simulink model "Model_leis_de_Newton"  (R2018a)
settings: Solver=FixedStepAuto  StartTime=0.0  StopTime=130  FixedStep=0.001  RelTol=1e-3
values from neighbouring files (symbols this model uses):
  C = [1 0 0 0 ... (first row only)    [Dados.m]    (also in Dados_correct.m; Function_ARE.m = D; teste.m = D)
  c = 0.0076    [Dados.m]    (also in Dados_correct.m; Function_ARE.m; areklmn_reactor.m; fd0.m)
  g = 9.81    [Dados.m]    (also in Dados_correct.m; Function_ARE.m; areklmn_reactor.m; fd0.m)
  Jphi = 0.00201    [Dados.m]    (also in Dados_correct.m; Function_ARE.m; areklmn_reactor.m; fd0.m)
  Jteta = 0.005425    [Dados.m]    (also in Dados_correct.m; Function_ARE.m; areklmn_reactor.m; fd0.m)
  K1 = Kpi(:,1:4)    [Dados.m]    (also in Dados_correct.m = Kpi90(:,1:4); Function_ARE.m = K(:,1:4); teste.m = K(:,1:4))
  K1_30 = Kpi30(:,1:4)    [Dados_correct.m]
  K2 = Kpi(:,5:6)    [Dados.m]    (also in Dados_correct.m = Kpi90(:,5:6); Function_ARE.m = K(:,5:6); teste.m = K(:,5:6))
  K2_30 = Kpi30(:,5:6)    [Dados_correct.m]
  Kf = 0.0275    [Dados.m]    (also in Dados_correct.m = 0.06; Function_ARE.m = 0.056; areklmn_reactor.m = 0.056; fd0.m = 0.056)
  L1 = 0.3    [Dados.m]    (also in Dados_correct.m = 0.227; Function_ARE.m = 0.227; areklmn_reactor.m = 0.227; fd0.m = 0.227)
  L2 = 0.1    [Dados.m]    (also in Dados_correct.m = 0.08; Function_ARE.m = 0.08; areklmn_reactor.m = 0.08; fd0.m = 0.08)
  Lw = 0.13    [Dados_correct.m]    (also in Function_ARE.m = 0.15; areklmn_reactor.m = 0.15; fd0.m = 0.15; teste.m = 0.15)
  Mh = 0.08    [Dados.m]    (also in Dados_correct.m; Function_ARE.m; areklmn_reactor.m; fd0.m)
  Mw = 0.08    [Dados_correct.m]    (also in Function_ARE.m = 0.039; areklmn_reactor.m = 0.039; fd0.m = 0.039; teste.m = 0.039)
undefined symbols (not defined in the file or in its folder): DiscIntNeverNeededParam, K1_130, K1_150, K1_90, K2_130, K2_150, K2_90, sigbuilder_block
settings Model: Creator=stayn  LastModifiedBy=stayn

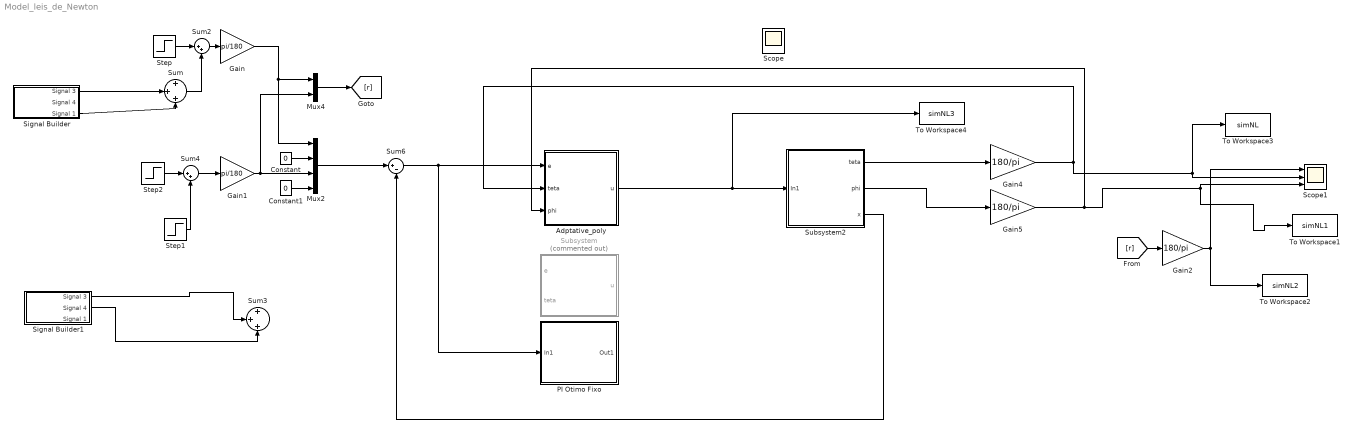
== system Model_leis_de_Newton ==
  Adptative_poly : Subsystem
  Constant : Constant  Value=0
  Constant1 : Constant  Value=0
  Gain : Gain  Gain=pi/180
  Gain1 : Gain  Gain=pi/180
  Gain2 : Gain  Gain=180/pi
  Gain4 : Gain  Gain=180/pi
  Gain5 : Gain  Gain=180/pi
  Mux2 : Mux
  Mux4 : Mux  Inputs=2
  PI Otimo Fixo : Subsystem
  Scope : Scope  NumInputPorts=2
  Scope1 : Scope  NumInputPorts=3
  Signal Builder : Subsystem  Tag=STV Subsys  LoadFcn=sigbuilder_block('load');  StartFcn=sigbuilder_block('start');  StopFcn=sigbuilder_block('stop');  ClipboardFcn=sigbuilder_block('clipboard');  mask(Sigbuilder block){tuvar=[0:10]}
      mask help: Simulink:masks:SigbuilderBlock_MD
      mask init:
      | if ~strcmp(get_param(bdroot(gcbh),'SimulationStatus'),'stopped') tuvar = sigbuilder_block('maskInit'); end
      settings: CopyFcn=sigbuilder_block('copy');  DeleteFcn=sigbuilder_block('delete');  ModelCloseFcn=sigbuilder_block('modelClose');  PreSaveFcn=sigbuilder_block('preSave');  PauseFcn=sigbuilder_block('pause');  ContinueFcn=sigbuilder_block('continue');  NameChangeFcn=sigbuilder_block('namechange');  OpenFcn=sigbuilder_block('open',[6 30 1012.5 447.75 ]);  CloseFcn=sigbuilder_block('close');
      mask Display: plot(0, 0, 100, 100,[2, 2, 32, 32, 2], [68, 8, 8, 68, 68],[32, 2], [38, 38], [32, 19, 2],[53, 60, 44], [32, 17, 17, 2],[16, 16, 31, 31]);txt = getActiveGroup(gcbh);text(2, 100, txt,'verticalAlignment', 'top');
  Signal Builder1 : Subsystem  Tag=STV Subsys  LoadFcn=sigbuilder_block('load');  StartFcn=sigbuilder_block('start');  StopFcn=sigbuilder_block('stop');  ClipboardFcn=sigbuilder_block('clipboard');  mask(Sigbuilder block){tuvar=[0:10]}
      mask help: Simulink:masks:SigbuilderBlock_MD
      mask init:
      | if ~strcmp(get_param(bdroot(gcbh),'SimulationStatus'),'stopped') tuvar = sigbuilder_block('maskInit'); end
      settings: CopyFcn=sigbuilder_block('copy');  DeleteFcn=sigbuilder_block('delete');  ModelCloseFcn=sigbuilder_block('modelClose');  PreSaveFcn=sigbuilder_block('preSave');  PauseFcn=sigbuilder_block('pause');  ContinueFcn=sigbuilder_block('continue');  NameChangeFcn=sigbuilder_block('namechange');  OpenFcn=sigbuilder_block('open',[6 30 1006.5 447.75 ]);  CloseFcn=sigbuilder_block('close');
      mask Display: plot(0, 0, 100, 100,[2, 2, 32, 32, 2], [68, 8, 8, 68, 68],[32, 2], [38, 38], [32, 19, 2],[53, 60, 44], [32, 17, 17, 2],[16, 16, 31, 31]);txt = getActiveGroup(gcbh);text(2, 100, txt,'verticalAlignment', 'top');
  Step : Step  Time=0  After=90  SampleTime=0
  Step1 : Step  Time=120  After=-20  SampleTime=0
  Step2 : Step  Time=100  After=30  SampleTime=0
  Subsystem : Subsystem  Commented=on
  Subsystem2 : Subsystem
  Sum : Sum  Inputs=+|+|+
  Sum2 : Sum  Inputs=|++
  Sum3 : Sum  Inputs=+|+|+
  Sum4 : Sum  Inputs=|++
  Sum6 : Sum  Inputs=|+-
  To Workspace1 : ToWorkspace  VariableName=simNL1  SampleTime=0.001
      settings: Save2DSignal=2-D array (concatenate along first dimension)
  To Workspace2 : ToWorkspace  VariableName=simNL2  SampleTime=0.001
      settings: Save2DSignal=2-D array (concatenate along first dimension)
  To Workspace3 : ToWorkspace  VariableName=simNL  SaveFormat=Structure With Time  SampleTime=0.001
      settings: Save2DSignal=2-D array (concatenate along first dimension)
  To Workspace4 : ToWorkspace  VariableName=simNL3  SampleTime=0.001
      settings: Save2DSignal=2-D array (concatenate along first dimension)
  wires:
  Subsystem2/3("x ") -> Sum6/2
  Sum6/1 -> PI Otimo Fixo/1(In1), Adptative_poly/1(e)
  Subsystem2/1("teta ") -> Gain4/1
  Signal Builder1/2(Signal 4) -> Sum3/3
  Sum4/1 -> Gain1/1
  Step2/1 -> Sum4/1
  Signal Builder1/1(Signal 3) -> Sum3/2
  Signal Builder/1(Signal 3) -> Sum/2
  Step/1 -> Sum2/1
  Mux2/1 -> Sum6/1
  Sum2/1 -> Gain/1
  Mux4/1 -> [r]
  Constant/1 -> Mux2/2
  Gain1/1 -> Mux4/2, Mux2/3
  Gain/1 -> Mux2/1, Mux4/1
  Constant1/1 -> Mux2/4
  [r] -> Gain2/1
  Signal Builder/3(Signal 1) -> Sum/3
  Gain2/1 -> To Workspace2/1, Scope1/1
  Gain5/1 -> Adptative_poly/3("phi "), To Workspace1/1, Scope1/3
  Subsystem2/2(phi) -> Gain5/1
  Gain4/1 -> To Workspace3/1, Scope1/2, Adptative_poly/2(teta)
  Adptative_poly/1(u) -> To Workspace4/1, Subsystem2/1(In1)
  Step1/1 -> Sum4/2
  Sum/1 -> Sum2/2

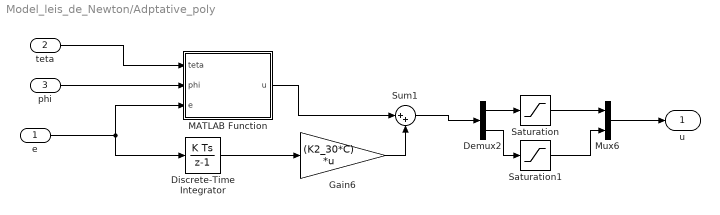
== system Model_leis_de_Newton/Adptative_poly ==
  e : Inport
  teta : Inport  Port=2
  "phi " : Inport  Port=3
  Demux2 : Demux  Outputs=2
  Discrete-Time Integrator : DiscreteIntegrator  SampleTime=0.001  ICPrevOutput=DiscIntNeverNeededParam  ICPrevScaledInput=DiscIntNeverNeededParam
  Gain6 : Gain  Gain=(K2_30*C)  Multiplication=Matrix(K*u) (u vector)
  MATLAB Function : MATLAB Function  TreatAsAtomicUnit=on
  Mux6 : Mux  Inputs=2
  Saturation : Saturate  UpperLimit=10  LowerLimit=0
  Saturation1 : Saturate  UpperLimit=5  LowerLimit=-5
  Sum1 : Sum  Inputs=|++
  u : Outport
  wires:
  MATLAB Function/1(u) -> Sum1/1
  e/1 -> Discrete-Time Integrator/1, MATLAB Function/3(e)
  Demux2/1 -> Saturation/1
  Saturation1/1 -> Mux6/2
  Demux2/2 -> Saturation1/1
  Discrete-Time Integrator/1 -> Gain6/1
  Gain6/1 -> Sum1/2
  teta/1 -> MATLAB Function/1(teta)
  Sum1/1 -> Demux2/1
  Saturation/1 -> Mux6/1
  Mux6/1 -> u/1
  "phi "/1 -> MATLAB Function/2(phi)

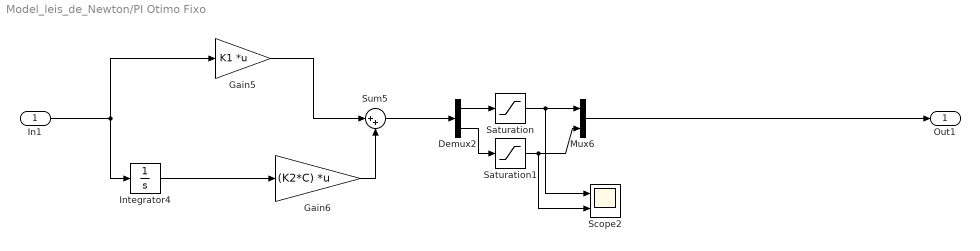
== system Model_leis_de_Newton/PI Otimo Fixo ==
  In1 : Inport
  Demux2 : Demux  Outputs=2
  Gain5 : Gain  Gain=K1  Multiplication=Matrix(K*u) (u vector)
  Gain6 : Gain  Gain=(K2*C)  Multiplication=Matrix(K*u) (u vector)
  Integrator4 : Integrator
  Mux6 : Mux  Inputs=2
  Saturation : Saturate  UpperLimit=10  LowerLimit=0
  Saturation1 : Saturate  UpperLimit=5  LowerLimit=-5
  Scope2 : Scope  NumInputPorts=2
  Sum5 : Sum  Inputs=|++
  Out1 : Outport
  wires:
  Saturation/1 -> Scope2/1, Mux6/1
  Integrator4/1 -> Gain6/1
  Demux2/1 -> Saturation/1
  Gain6/1 -> Sum5/2
  In1/1 -> Gain5/1, Integrator4/1
  Gain5/1 -> Sum5/1
  Saturation1/1 -> Mux6/2, Scope2/2
  Demux2/2 -> Saturation1/1
  Sum5/1 -> Demux2/1
  Mux6/1 -> Out1/1

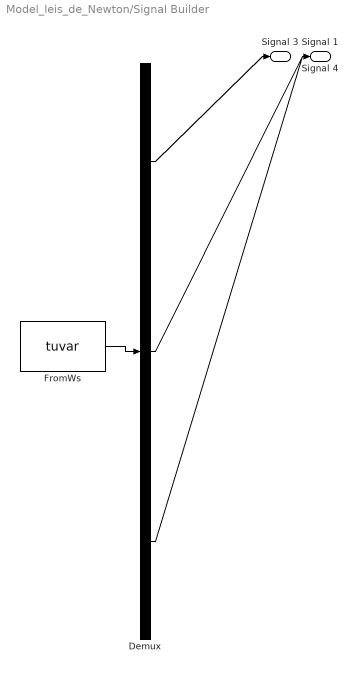
== system Model_leis_de_Newton/Signal Builder ==
  Demux : Demux  Tag=STV Demux  Outputs=3
  FromWs : FromWorkspace  Tag=STV FromWs  VariableName=tuvar  SampleTime=0
      SigBuilderData=|
      | common.afterFinalStr = 'Extrapolate'
      | common.sampleTime = 0
      | dataSet.timeRange = [0 100]
      | dataSet.name = 'Group 1'
      | sbobj.Groups.Name = 'Group 1'
      | sbobj.Groups.Signals(1).Name = 'Signal 3'
      | sbobj.Groups.Signals(1).XData = [0 20 20 45 45 100]
      | sbobj.Groups.Signals(1).YData = [0 0 45 45 0 0]
      | sbobj.Groups.Signals(2).Name = 'Signal 4'
      | sbobj.Groups.Signals(2).XData = [0 65 65 100]
      | sbobj.Groups.Signals(2).YData = [0 0 -35 -35]
      | sbobj.Groups.Signals(3).Name = 'Signal 1'
      | sbobj.Groups.Signals(3).XData = [0 65 65 85 85 100]
      | sbobj.Groups.Signals(3).YData = [0 0 -30 -30 0 0]
      | sbobj.Groups.TimeRange = [0 100]
  Signal 3 : Outport  Tag=STV Outport
  Signal 4 : Outport  Tag=STV Outport  Port=2
  Signal 1 : Outport  Tag=STV Outport  Port=3
  wires:
  FromWs/1 -> Demux/1
  Demux/1 -> Signal 3/1
  Demux/2 -> Signal 4/1
  Demux/3 -> Signal 1/1

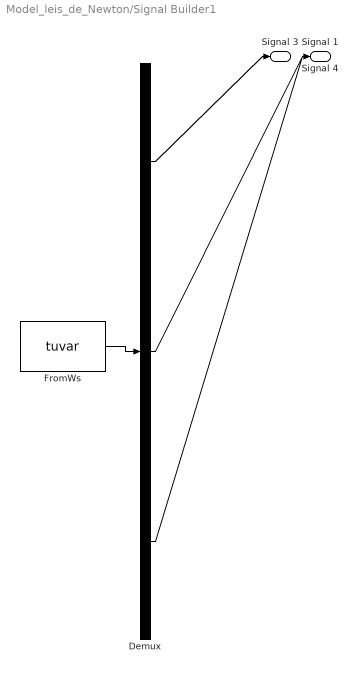
== system Model_leis_de_Newton/Signal Builder1 ==
  Demux : Demux  Tag=STV Demux  Outputs=3
  FromWs : FromWorkspace  Tag=STV FromWs  VariableName=tuvar  SampleTime=0
      SigBuilderData=|
      | common.afterFinalStr = 'Extrapolate'
      | common.sampleTime = 0
      | dataSet.timeRange = [0 100]
      | dataSet.name = 'Group 1'
      | sbobj.Groups.Name = 'Group 1'
      | sbobj.Groups.Signals(1).Name = 'Signal 3'
      | sbobj.Groups.Signals(1).XData = [0 15.1 15.1 30.1 30.1 100]
      | sbobj.Groups.Signals(1).YData = [0 0 -45 -45 0 0]
      | sbobj.Groups.Signals(2).Name = 'Signal 4'
      | sbobj.Groups.Signals(2).XData = [0 45 45 60 60 100]
      | sbobj.Groups.Signals(2).YData = [0 0 40 40 0 0]
      | sbobj.Groups.Signals(3).Name = 'Signal 1'
      | sbobj.Groups.Signals(3).XData = [0 70.1 70.1 85.6 85.6 100]
      | sbobj.Groups.Signals(3).YData = [0 0 50.5 50.5 0 0]
      | sbobj.Groups.TimeRange = [0 100]
  Signal 3 : Outport  Tag=STV Outport
  Signal 4 : Outport  Tag=STV Outport  Port=2
  Signal 1 : Outport  Tag=STV Outport  Port=3
  wires:
  FromWs/1 -> Demux/1
  Demux/1 -> Signal 3/1
  Demux/2 -> Signal 4/1
  Demux/3 -> Signal 1/1

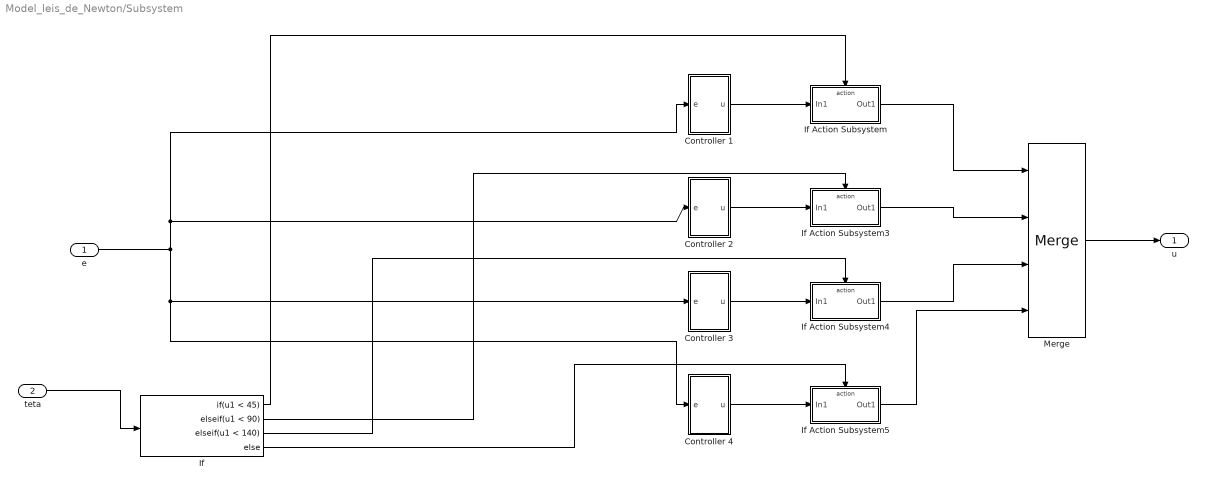
== system Model_leis_de_Newton/Subsystem ==
  e : Inport
  teta : Inport  Port=2
  Controller 1 : Subsystem
  Controller 2 : Subsystem
  Controller 3 : Subsystem
  Controller 4 : Subsystem
  If : If  IfExpression=u1 < 45  ElseIfExpressions=u1 < 90, u1 < 140
  If Action Subsystem : Subsystem  TreatAsAtomicUnit=on
  If Action Subsystem3 : Subsystem  TreatAsAtomicUnit=on
  If Action Subsystem4 : Subsystem  TreatAsAtomicUnit=on
  If Action Subsystem5 : Subsystem  TreatAsAtomicUnit=on
  Merge : Merge  Inputs=4
  u : Outport
  wires:
  Controller 3/1("u ") -> If Action Subsystem4/1(In1)
  Controller 1/1("u ") -> If Action Subsystem/1(In1)
  e/1 -> Controller 1/1("e "), Controller 2/1("e "), Controller 4/1("e "), Controller 3/1("e ")
  If Action Subsystem4/1(Out1) -> Merge/3
  teta/1 -> If/1
  Merge/1 -> u/1
  Controller 4/1("u ") -> If Action Subsystem5/1(In1)
  If Action Subsystem/1(Out1) -> Merge/1
  Controller 2/1("u ") -> If Action Subsystem3/1(In1)
  If Action Subsystem3/1(Out1) -> Merge/2
  If Action Subsystem5/1(Out1) -> Merge/4
  If/1 -> If Action Subsystem/Action
  If/2 -> If Action Subsystem3/Action
  If/3 -> If Action Subsystem4/Action
  If/4 -> If Action Subsystem5/Action

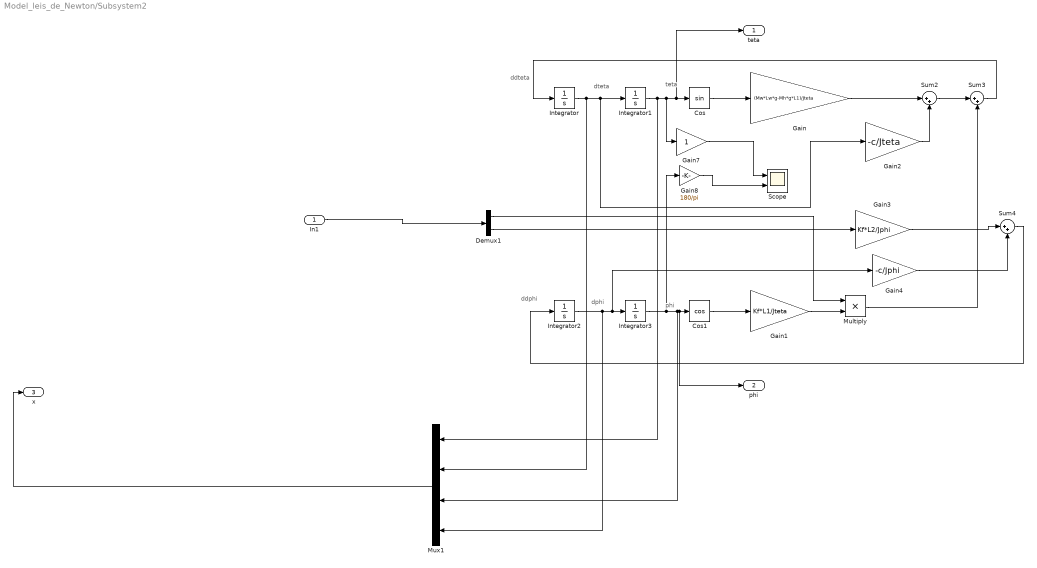
== system Model_leis_de_Newton/Subsystem2 ==
  note: ddphi
  note: phi
  note: dphi
  note: teta
  note: dteta
  note: ddteta
  In1 : Inport
  Cos : Trigonometry
  Cos1 : Trigonometry  Operator=cos
  Demux1 : Demux  Outputs=2
  Gain : Gain  Gain=(Mw*Lw*g-Mh*g*L1)/Jteta
  Gain1 : Gain  Gain=Kf*L1/Jteta
  Gain2 : Gain  Gain=-c/Jteta
  Gain3 : Gain  Gain=Kf*L2/Jphi
  Gain4 : Gain  Gain=-c/Jphi
  Gain7 : Gain
  Gain8 : Gain  Gain=180/pi
  Integrator{,1..3} (4 alike) : Integrator
  Multiply : Product
  Mux1 : Mux
  Scope : Scope  NumInputPorts=2
  Sum2 : Sum  Inputs=|++
  Sum3 : Sum  Inputs=|++
  Sum4 : Sum  Inputs=|++
  "teta " : Outport
  phi : Outport  Port=2
  "x " : Outport  Port=3
  wires:
  Integrator2/1 -> Mux1/4, Gain4/1, Integrator3/1
  Integrator3/1 -> Gain8/1, Mux1/3, phi/1, Cos1/1
  Integrator/1 -> Mux1/2, Gain2/1, Integrator1/1
  Demux1/1 -> Multiply/1
  Cos1/1 -> Gain1/1
  Sum3/1 -> Integrator/1
  Integrator1/1 -> Mux1/1, Gain7/1, "teta "/1, Cos/1
  Gain4/1 -> Sum4/2
  Demux1/2 -> Gain3/1
  Gain/1 -> Sum2/1
  Sum2/1 -> Sum3/1
  Gain3/1 -> Sum4/1
  Gain2/1 -> Sum2/2
  Gain7/1 -> Scope/1
  Gain8/1 -> Scope/2
  Gain1/1 -> Multiply/2
  Cos/1 -> Gain/1
  Sum4/1 -> Integrator2/1
  Multiply/1 -> Sum3/2
  Mux1/1 -> "x "/1
  In1/1 -> Demux1/1

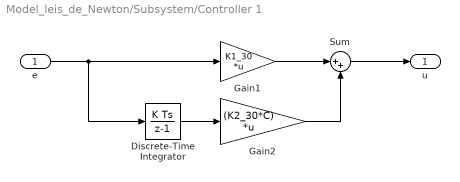
== system Model_leis_de_Newton/Subsystem/Controller 1 ==
  "e " : Inport
  Discrete-Time Integrator : DiscreteIntegrator  SampleTime=0.025  ICPrevOutput=DiscIntNeverNeededParam  ICPrevScaledInput=DiscIntNeverNeededParam
  Gain1 : Gain  Gain=K1_30  Multiplication=Matrix(K*u) (u vector)
  Gain2 : Gain  Gain=(K2_30*C)  Multiplication=Matrix(K*u) (u vector)
  Sum : Sum  Inputs=|++
  "u " : Outport
  wires:
  Discrete-Time Integrator/1 -> Gain2/1
  "e "/1 -> Discrete-Time Integrator/1, Gain1/1
  Gain1/1 -> Sum/1
  Gain2/1 -> Sum/2
  Sum/1 -> "u "/1

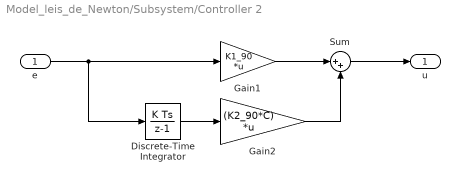
== system Model_leis_de_Newton/Subsystem/Controller 2 ==
  "e " : Inport
  Discrete-Time Integrator : DiscreteIntegrator  SampleTime=0.025  ICPrevOutput=DiscIntNeverNeededParam  ICPrevScaledInput=DiscIntNeverNeededParam
  Gain1 : Gain  Gain=K1_90  Multiplication=Matrix(K*u) (u vector)
  Gain2 : Gain  Gain=(K2_90*C)  Multiplication=Matrix(K*u) (u vector)
  Sum : Sum  Inputs=|++
  "u " : Outport
  wires:
  Discrete-Time Integrator/1 -> Gain2/1
  "e "/1 -> Discrete-Time Integrator/1, Gain1/1
  Gain1/1 -> Sum/1
  Gain2/1 -> Sum/2
  Sum/1 -> "u "/1

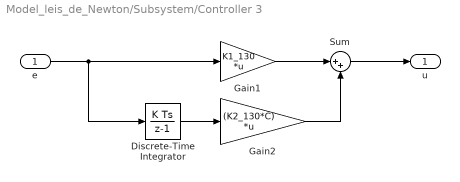
== system Model_leis_de_Newton/Subsystem/Controller 3 ==
  "e " : Inport
  Discrete-Time Integrator : DiscreteIntegrator  SampleTime=0.025  ICPrevOutput=DiscIntNeverNeededParam  ICPrevScaledInput=DiscIntNeverNeededParam
  Gain1 : Gain  Gain=K1_130  Multiplication=Matrix(K*u) (u vector)
  Gain2 : Gain  Gain=(K2_130*C)  Multiplication=Matrix(K*u) (u vector)
  Sum : Sum  Inputs=|++
  "u " : Outport
  wires:
  Discrete-Time Integrator/1 -> Gain2/1
  "e "/1 -> Discrete-Time Integrator/1, Gain1/1
  Gain1/1 -> Sum/1
  Gain2/1 -> Sum/2
  Sum/1 -> "u "/1

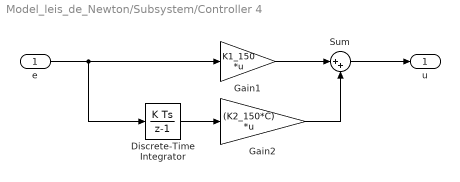
== system Model_leis_de_Newton/Subsystem/Controller 4 ==
  "e " : Inport
  Discrete-Time Integrator : DiscreteIntegrator  SampleTime=0.025  ICPrevOutput=DiscIntNeverNeededParam  ICPrevScaledInput=DiscIntNeverNeededParam
  Gain1 : Gain  Gain=K1_150  Multiplication=Matrix(K*u) (u vector)
  Gain2 : Gain  Gain=(K2_150*C)  Multiplication=Matrix(K*u) (u vector)
  Sum : Sum  Inputs=|++
  "u " : Outport
  wires:
  Discrete-Time Integrator/1 -> Gain2/1
  "e "/1 -> Discrete-Time Integrator/1, Gain1/1
  Gain1/1 -> Sum/1
  Gain2/1 -> Sum/2
  Sum/1 -> "u "/1

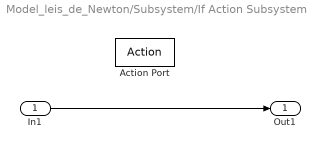
== system Model_leis_de_Newton/Subsystem/If Action Subsystem ==
  In1 : Inport
  Action Port : ActionPort  PropagateVarSize=During execution  ActionType=then
  Out1 : Outport
  wires:
  In1/1 -> Out1/1

== system Model_leis_de_Newton/Subsystem/If Action Subsystem3 ==
  In1 : Inport
  Action Port : ActionPort  PropagateVarSize=During execution  ActionType=elseif
  Out1 : Outport
  wires:
  In1/1 -> Out1/1

== system Model_leis_de_Newton/Subsystem/If Action Subsystem4 ==
  In1 : Inport
  Action Port : ActionPort  PropagateVarSize=During execution  ActionType=elseif
  Out1 : Outport
  wires:
  In1/1 -> Out1/1

== system Model_leis_de_Newton/Subsystem/If Action Subsystem5 ==
  In1 : Inport
  Action Port : ActionPort  PropagateVarSize=During execution  ActionType=else
  Out1 : Outport
  wires:
  In1/1 -> Out1/1

== matlab function Model_leis_de_Newton/Adptative_poly/MATLAB Function ==
  settings: updateMethod=DISCRETE
  data: teta input; phi input; u output; e input
 function u = fcn(teta,phi,e)
x = phi;
y= teta;
persistent K1;
isempty(K1)
    pp00 =  1.792; pp01 = 0.05293; pp02 =  -4.347e-05;
    pp20 = -0.003316; pp21 = -2.997e-05; pp22 = 4.784e-07;
    pp40 =5.41e-07;
    p00 = 1.275; p01 = 0.001739; p02 = 2.001e-05;  
    p20 = -0.001137; p21 = 3.313e-06; p22 = 5.662e-08;  
    p40 = 1.397e-07;
   
    K1 = [0.345552654675701 0.207922866674390 1.52365480300072e-16 1.41750121698813e-17;
          2.34353074450996e-17 1.34831465617473e-17 3.19016248053525 0.692343603732364];
    
K1(1,1) = pp00 + pp01*y + pp20*x^2 + pp02*y^2 + pp21*x^2*y + pp40*x^4 + pp22*x^2*y^2;
K1(1,2) = p00 + p01*y + p20*x^2 + p02*y^2 + p21*x^2*y + p40*x^4 + p22*x^2*y^2;

u = K1*e;
